simulink model "product_dma"  (R2020a)
settings: Solver=VariableStepAuto  StartTime=0.0  StopTime=10.0  RelTol=1e-3
settings Model: Creator=sunip  LastModifiedBy=sunip

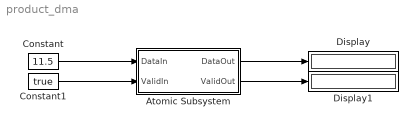
== system product_dma ==
  Atomic Subsystem : Subsystem  TreatAsAtomicUnit=on
  Constant : Constant  Value=11.5  OutDataTypeStr=single
  Constant1 : Constant  Value=true
  Display : Display
  Display1 : Display
  wires:
  Constant/1 -> Atomic Subsystem/1(DataIn)
  Constant1/1 -> Atomic Subsystem/2(ValidIn)
  Atomic Subsystem/1(DataOut) -> Display/1
  Atomic Subsystem/2(ValidOut) -> Display1/1

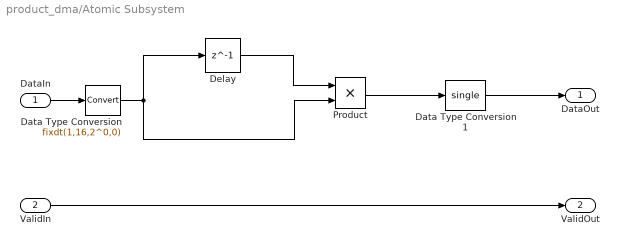
== system product_dma/Atomic Subsystem ==
  DataIn : Inport  OutDataTypeStr=single
  ValidIn : Inport  Port=2  OutDataTypeStr=boolean
  Data Type Conversion : DataTypeConversion  OutDataTypeStr=fixdt(1,16,2^0,0)  RndMeth=Round
  Data Type Conversion1 : DataTypeConversion  OutDataTypeStr=single
  Delay : Delay  DelayLength=1
  Product : Product
  DataOut : Outport  OutDataTypeStr=single
  ValidOut : Outport  Port=2  OutDataTypeStr=boolean
  wires:
  DataIn/1 -> Data Type Conversion/1
  Delay/1 -> Product/1
  Data Type Conversion/1 -> Product/2, Delay/1
  Product/1 -> Data Type Conversion1/1
  Data Type Conversion1/1 -> DataOut/1
  ValidIn/1 -> ValidOut/1
